simulink model "problem5"  (R2020b)
settings: Solver=VariableStepAuto  StartTime=0.0  StopTime=0.01  MaxStep=0.0001  RelTol=1e-3
settings Model: Creator=ARPITA  LastModifiedBy=ARPITA

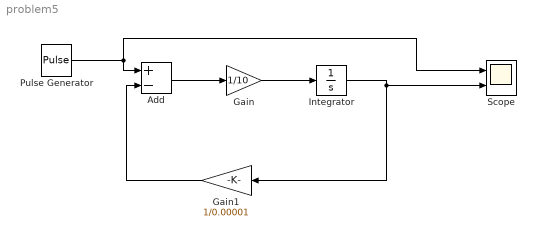
== system problem5 ==
  Add : Sum  Inputs=+-
  Gain : Gain  Gain=1/10
  Gain1 : Gain  Gain=1/0.00001
  Integrator : Integrator  InitialCondition=2
  Pulse Generator : DiscretePulseGenerator  PulseType=Time based  Period=0.01  PulseWidth=2
  Scope : Scope  NumInputPorts=2
  wires:
  Add/1 -> Gain/1
  Gain/1 -> Integrator/1
  Gain1/1 -> Add/2
  Integrator/1 -> Scope/2, Gain1/1
  Pulse Generator/1 -> Add/1, Scope/1
